simulink model "teste"  (R2015a)
settings: Solver=ode45  StartTime=0.0  StopTime=10.0  RelTol=1e-3
values from neighbouring files (symbols this model uses):
  Ts = 1/fs    (= 0.05)    [ex6.m]    (also in sim_ex6.m = C.Ts)
settings Model: Creator=brunopeixoto  LastModifiedBy=brunopeixoto

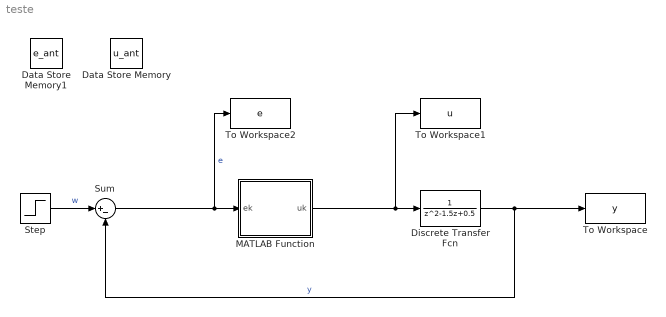
== system teste ==
  Data Store Memory : DataStoreMemory  DataStoreName=u_ant  ReadBeforeWriteMsg=warning  WriteAfterWriteMsg=warning  WriteAfterReadMsg=warning  OutDataTypeStr=double
  Data Store Memory1 : DataStoreMemory  DataStoreName=e_ant  ReadBeforeWriteMsg=warning  WriteAfterWriteMsg=warning  WriteAfterReadMsg=warning  InitialValue=[0, 0]  OutDataTypeStr=double
  Discrete Transfer Fcn : DiscreteTransferFcn  Denominator=[1 -1.5 0.5]
  MATLAB Function : MATLAB Function  TreatAsAtomicUnit=on
  Step : Step  Time=0  SampleTime=Ts
  Sum : Sum  Inputs=|+-
  To Workspace : ToWorkspace  VariableName=y  SaveFormat=Structure With Time  SampleTime=-1
  To Workspace1 : ToWorkspace  VariableName=u  SaveFormat=Structure With Time  SampleTime=-1
  To Workspace2 : ToWorkspace  VariableName=e  SaveFormat=Structure With Time  SampleTime=-1
  wires:
  Step/1 -> Sum/1  "w"
  Discrete Transfer Fcn/1 -> To Workspace/1, Sum/2  "y"
  MATLAB Function/1(uk) -> Discrete Transfer Fcn/1, To Workspace1/1
  Sum/1 -> To Workspace2/1, MATLAB Function/1(ek)  "e"

== matlab function teste/MATLAB Function ==
  data: ek input; uk output; e_ant data_store_memory; u_ant data_store_memory
% @author: Bruno Peixoto
% Efetua o controle de posicao de um motor DC
% por transformacao de tustin
function uk = controlador(ek)
    global u_ant;
    
    b = 0.5;
    K = 0.0625;
    
    % Acao de controle
     uk = K*ek;

    % Atualizacao da acao de controle
    u_ant = uk; 
end
